simulink model "model_5LinkWalking"  (R2022b)
settings: Solver=ode45  StartTime=0.0  StopTime=Tf  FixedStep=1e-5  MaxStep=1e-3  RelTol=1e-12  AbsTol=1e-8
values from neighbouring files (symbols this model uses):
  des_traj_alpha = [ ... (first row only)    [main.m]
  f_dist = [0; -100; 0]    [main.m]
  gains = [ ... (first row only)    [main.m]
  gains_VSLIPSL = [gain_VSLIPSL.K_p; gain_VSLIPSL.K_d; gain_VSLIPSL.K_p_sw; gain_VSLIPSL.K_d_sw; gain_VSLIPSL.K_p_ds; gain_VSLIPSL.K_d_ds; gain_VSLIPSL.K_v_ds]    [main.m]
  init_flag = [1; 0; -dc.col_param.footPlus; -slipsl.time_ss(N); slipsl.x_ss(1); slipsl.y_ss(1); alpha_ss_ref(1)]    [main.m]
  Initial_state = [q0;dq0]    [main.m]
  param = [ ... (first row only)    [main.m]
  ref_star_ds = [ref_star.ds.x_CoM_star,      ref_star.ds.y_CoM_star, ref_star.ds.dx_CoM_star,      ref_star.ds.del_y_CoM_star, ref_star.ds.del_dx_CoM_star,      ref_star.ds.del2_y_CoM_star]    [main.m]
  ref_star_ss = [ref_star.ss.x_M_star,      ref_star.ss.y_M_star, ref_star.ss.x_swFoot_star, ref_star.ss.y_swFoot_star,      ref_star.ss.del_y_M_star, ref_star.ss.del_x_swFoot_star, ref_star.ss.del_y_swFoot_star,      ref_star.ss.del2_y_M_star, ref_star.ss.del2_x_swFoot_star, ref_star.ss.del2_y_swFoot_star,      ref_star.ss.x_CoM_star]    [main.m]
  sample_time = 0.001    [main.m]
  slipslParams = [ ... (first row only)    [main.m]
  slipslTraj_ds = [slipsl.time_ds, slipsl.x_ds, slipsl.y_ds, slipsl.dx_ds, slipsl.dy_ds, alpha_ds_ref_discrete]    [main.m]
  slipslTraj_ss = [slipsl.time_ss, slipsl.x_ss, slipsl.y_ss, slipsl.dx_ss, slipsl.dy_ss, alpha_ss_ref_discrete]    [main.m]
  swFootTraj = [swFootSLIPSL.x_CoM, swFootSLIPSL.x, swFootSLIPSL.z, swFootSLIPSL.dx, swFootSLIPSL.dz]    [main.m]
undefined symbols (not defined in the file or in its folder): sim_settings
libraries: simulink x1
(part 1 of 2)
settings Model: Creator=yamakita_lab  LastModifiedBy=mmpel
settings SolverCC: AutoScaleAbsTol=off  AlgebraicLoopSolver=TrustRegion
settings DataIOCC: ReturnWorkspaceOutputs=off
settings DebuggingCC: UnconnectedInputMsg=warning  UnconnectedOutputMsg=warning  UnconnectedLineMsg=warning  SFMachineParentedDataDiag=warning  ArithmeticOperatorsInVariantConditions=warning
settings ModelReferenceCC: EnableRefExpFcnMdlSchedulingChecks=on
settings SFSimCC: SimUseLocalCustomCode=off  CustomCodeUndefinedFunction=UseInterfaceOnly
settings RTWCC: RTWUseLocalCustomCode=off  DLArmComputeVersion=19.05

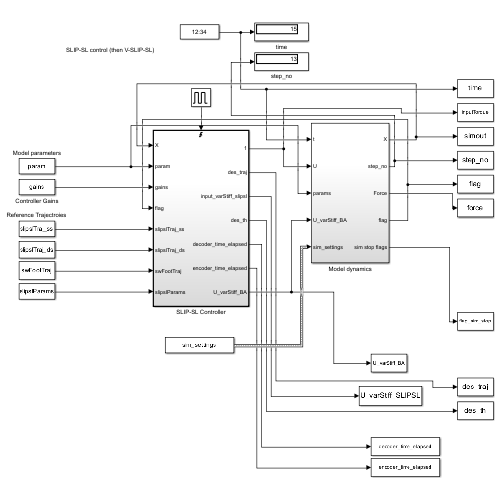
[thumbnail: Simulink's stored preview of the top-level diagram]
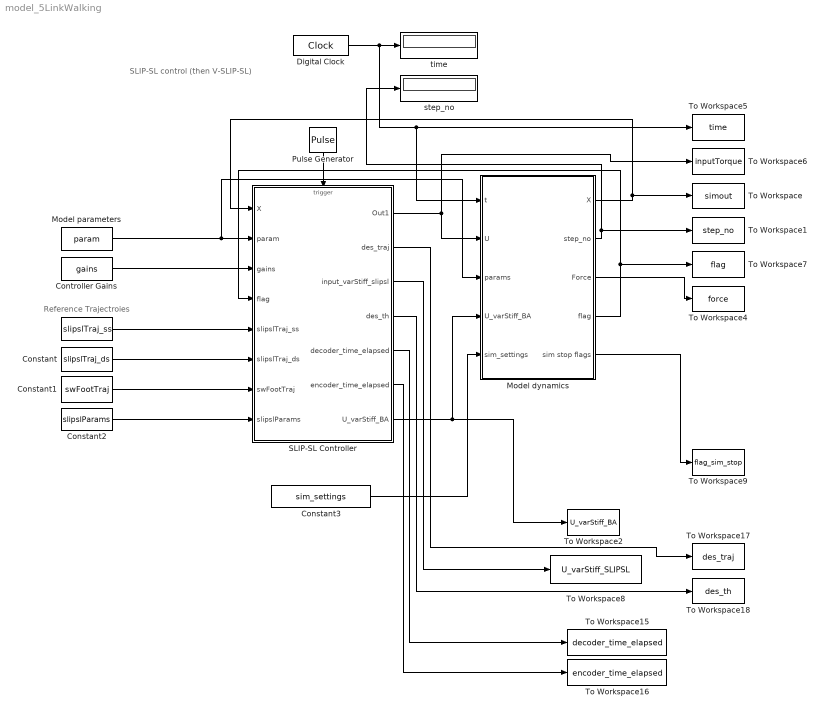
== system model_5LinkWalking ==
  note: Reference Trajectroies
  note: SLIP-SL control (then V-SLIP-SL)
  " " : Constant  Value=slipslTraj_ss
  Constant : Constant  Value=slipslTraj_ds
  Constant1 : Constant  Value=swFootTraj
  Constant2 : Constant  Value=slipslParams
  Constant3 : Constant  Value=sim_settings  VectorParams1D=off  OutDataTypeStr=Bus: sim_settings_bus
  Controller Gains : Constant  Value=gains
  Digital Clock : DigitalClock  SampleTime=1e-4
  Model dynamics : Subsystem
  Model parameters : Constant  Value=param  OutDataTypeStr=double
  Pulse Generator : DiscretePulseGenerator  PulseType=Time based  Period=5e-4  PulseWidth=5
  SLIP-SL Controller : Subsystem  TreatAsAtomicUnit=on
  To Workspace : ToWorkspace  VariableName=simout  SampleTime=sample_time
  To Workspace1 : ToWorkspace  VariableName=step_no  SampleTime=sample_time
  To Workspace15 : ToWorkspace  VariableName=decoder_time_elapsed  SampleTime=sample_time
  To Workspace16 : ToWorkspace  VariableName=encoder_time_elapsed  SampleTime=sample_time
  To Workspace17 : ToWorkspace  VariableName=des_traj  SampleTime=sample_time
  To Workspace18 : ToWorkspace  VariableName=des_th  SampleTime=sample_time
  To Workspace2 : ToWorkspace  VariableName=U_varStiff_BA  SampleTime=sample_time
  To Workspace4 : ToWorkspace  VariableName=force  SampleTime=sample_time
  To Workspace5 : ToWorkspace  VariableName=time  SampleTime=sample_time
  To Workspace6 : ToWorkspace  VariableName=inputTorque  SampleTime=sample_time
  To Workspace7 : ToWorkspace  VariableName=flag  SampleTime=sample_time
  To Workspace8 : ToWorkspace  VariableName=U_varStiff_SLIPSL  SampleTime=sample_time
  To Workspace9 : ToWorkspace  VariableName=flag_sim_stop  SampleTime=sample_time
  step_no : Display
  time : Display
  wires:
  SLIP-SL Controller/1(Out1) -> To Workspace6/1, Model dynamics/2(U)
  Model dynamics/1(X) -> SLIP-SL Controller/1(X), To Workspace/1
  Digital Clock/1 -> Model dynamics/1(t), To Workspace5/1, time/1
  Model dynamics/2(step_no) -> step_no/1, To Workspace1/1
  Model dynamics/3(Force) -> To Workspace4/1
  Model parameters/1 -> Model dynamics/3(params), SLIP-SL Controller/2(param)
  Controller Gains/1 -> SLIP-SL Controller/3(gains)
  Model dynamics/4(flag) -> To Workspace7/1, SLIP-SL Controller/4(flag)
  " "/1 -> SLIP-SL Controller/5(slipslTraj_ss)
  Constant1/1 -> SLIP-SL Controller/7(swFootTraj)
  Pulse Generator/1 -> SLIP-SL Controller/Trigger
  Model dynamics/5(sim stop flags) -> To Workspace9/1
  SLIP-SL Controller/3(input_varStiff_slipsl) -> To Workspace8/1
  SLIP-SL Controller/5(decoder_time_elapsed) -> To Workspace15/1
  SLIP-SL Controller/6(encoder_time_elapsed) -> To Workspace16/1
  SLIP-SL Controller/2(des_traj) -> To Workspace17/1
  SLIP-SL Controller/4(des_th) -> To Workspace18/1
  Constant/1 -> SLIP-SL Controller/6(slipslTraj_ds)
  Constant2/1 -> SLIP-SL Controller/8(slipslParams)
  SLIP-SL Controller/7(U_varStiff_BA) -> Model dynamics/4(U_varStiff_BA), To Workspace2/1
  Constant3/1 -> Model dynamics/5(sim_settings)

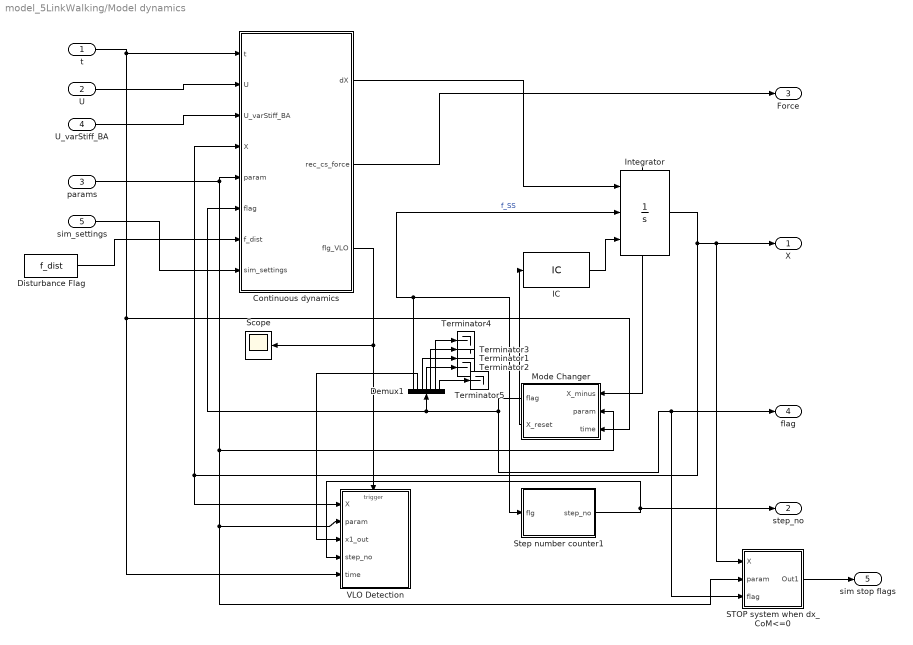
== system model_5LinkWalking/Model dynamics ==
  t : Inport
  U : Inport  Port=2
  params : Inport  Port=3
  U_varStiff_BA : Inport  Port=4
  sim_settings : Inport  Port=5
  Continuous dynamics : MATLAB Function  TreatAsAtomicUnit=on
  Demux1 : Demux  Outputs=7
  Disturbance Flag : Constant  Value=f_dist
  IC : InitialCondition  Value=Initial_state
  Integrator : Integrator  ExternalReset=falling  InitialConditionSource=external  ShowStatePort=on
  Mode Changer : Subsystem
  STOP system when dx_CoM<=0 : Subsystem
  Scope : Scope
  Step number counter1 : Subsystem
  Terminator{1..5} (5 alike) : Terminator
  VLO Detection : Subsystem  TreatAsAtomicUnit=on
  X : Outport  VectorParamsAs1DForOutWhenUnconnected=off
  step_no : Outport  Port=2  VectorParamsAs1DForOutWhenUnconnected=off
  Force : Outport  Port=3  VectorParamsAs1DForOutWhenUnconnected=off
  flag : Outport  Port=4
  sim stop flags : Outport  Port=5
  wires:
  IC/1 -> Integrator/3
  Integrator/State -> Mode Changer/1(X_minus)
  Continuous dynamics/1(dX) -> Integrator/1
  params/1 -> STOP system when dx_CoM<=0/2(param), VLO Detection/2(param), Mode Changer/2("param "), Continuous dynamics/5(param)
  U/1 -> Continuous dynamics/2(U)
  t/1 -> VLO Detection/5(time), Mode Changer/3(time), Continuous dynamics/1(t)
  Continuous dynamics/3(flg_VLO) -> Scope/1, VLO Detection/Trigger
  Integrator/1 -> STOP system when dx_CoM<=0/1(X), X/1, Continuous dynamics/4(X), VLO Detection/1(X)
  Mode Changer/2(X_reset) -> IC/1
  Mode Changer/1(flag) -> STOP system when dx_CoM<=0/3(flag), flag/1, Demux1/1, Continuous dynamics/6(flag)
  Demux1/2 -> VLO Detection/3(x1_out)
  Demux1/3 -> Terminator1/1
  Demux1/1 -> Step number counter1/1(flg), Integrator/2  "f_SS"
  Step number counter1/1(step_no) -> VLO Detection/4(step_no), step_no/1
  Continuous dynamics/2(rec_cs_force) -> Force/1
  Demux1/4 -> Terminator2/1
  Demux1/5 -> Terminator3/1
  Demux1/6 -> Terminator4/1
  STOP system when dx_CoM<=0/1(Out1) -> sim stop flags/1
  Disturbance Flag/1 -> Continuous dynamics/7(f_dist)
  Demux1/7 -> Terminator5/1
  U_varStiff_BA/1 -> Continuous dynamics/3(U_varStiff_BA)
  sim_settings/1 -> Continuous dynamics/8(sim_settings)

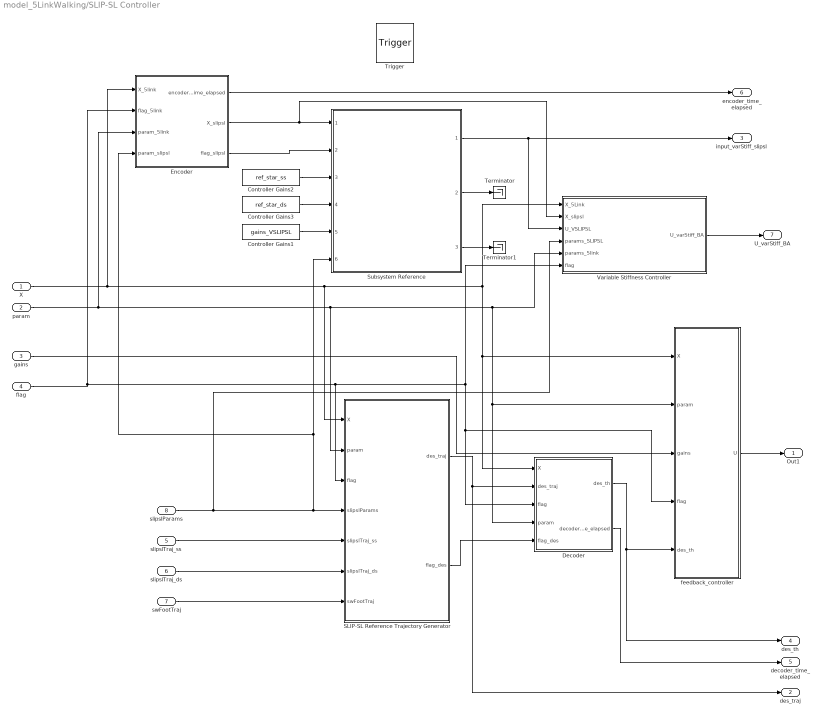
== system model_5LinkWalking/SLIP-SL Controller ==
  X : Inport
  param : Inport  Port=2
  gains : Inport  Port=3
  flag : Inport  Port=4
  slipslTraj_ss : Inport  Port=5
  slipslTraj_ds : Inport  Port=6
  swFootTraj : Inport  Port=7
  slipslParams : Inport  Port=8
  Trigger : TriggerPort  VariantControl=Variant  PortDimensions=1
  Controller Gains1 : Constant  Value=gains_VSLIPSL
  Controller Gains2 : Constant  Value=ref_star_ss
  Controller Gains3 : Constant  Value=ref_star_ds
  Decoder : MATLAB Function  TreatAsAtomicUnit=on
  Encoder : MATLAB Function  TreatAsAtomicUnit=on
  SLIP-SL Reference Trajectory Generator : MATLAB Function  TreatAsAtomicUnit=on
  Subsystem Reference : Subsystem  ReferencedSubsystem=VSLIPSL_controller_subsystem
  Terminator : Terminator
  Terminator1 : Terminator
  Variable Stiffness Controller : MATLAB Function  TreatAsAtomicUnit=on
  feedback_controller : MATLAB Function  TreatAsAtomicUnit=on
  Out1 : Outport  VectorParamsAs1DForOutWhenUnconnected=off
  des_traj : Outport  Port=2  InitialOutput=des_traj_alpha  VectorParamsAs1DForOutWhenUnconnected=off
  input_varStiff_slipsl : Outport  Port=3  VectorParamsAs1DForOutWhenUnconnected=off
  des_th : Outport  Port=4  PortDimensions=10  InitialOutput=Initial_state  VectorParamsAs1DForOutWhenUnconnected=off
  decoder_time_elapsed : Outport  Port=5  VectorParamsAs1DForOutWhenUnconnected=off
  encoder_time_elapsed : Outport  Port=6  VectorParamsAs1DForOutWhenUnconnected=off
  U_varStiff_BA : Outport  Port=7  VectorParamsAs1DForOutWhenUnconnected=off
  wires:
  feedback_controller/1(U) -> Out1/1
  X/1 -> SLIP-SL Reference Trajectory Generator/1(X), Variable Stiffness Controller/1(X_5Link), Decoder/1(X), feedback_controller/1(X), Encoder/1(X_5link)
  param/1 -> SLIP-SL Reference Trajectory Generator/2(param), Variable Stiffness Controller/5(params_5link), Decoder/4(param), feedback_controller/2(param), Encoder/3(param_5link)
  gains/1 -> feedback_controller/3(gains)
  flag/1 -> Encoder/2(flag_5link), Variable Stiffness Controller/6(flag), feedback_controller/4(flag), Decoder/3(flag), SLIP-SL Reference Trajectory Generator/3(flag)
  slipslTraj_ss/1 -> SLIP-SL Reference Trajectory Generator/5(slipslTraj_ss)
  swFootTraj/1 -> SLIP-SL Reference Trajectory Generator/7(swFootTraj)
  SLIP-SL Reference Trajectory Generator/1(des_traj) -> des_traj/1, Decoder/2(des_traj)
  slipslParams/1 -> Variable Stiffness Controller/4(params_SLIPSL), Encoder/4(param_slipsl), Subsystem Reference/6, SLIP-SL Reference Trajectory Generator/4(slipslParams)
  Controller Gains1/1 -> Subsystem Reference/5
  Controller Gains2/1 -> Subsystem Reference/3
  Controller Gains3/1 -> Subsystem Reference/4
  slipslTraj_ds/1 -> SLIP-SL Reference Trajectory Generator/6(slipslTraj_ds)
  Decoder/1(des_th) -> feedback_controller/5(des_th), des_th/1
  SLIP-SL Reference Trajectory Generator/2(flag_des) -> Decoder/5(flag_des)
  Decoder/2(decoder_time_elapsed) -> decoder_time_elapsed/1
  Encoder/2(X_slipsl) -> Variable Stiffness Controller/2(X_slipsl), Subsystem Reference/1
  Encoder/3(flag_slipsl) -> Subsystem Reference/2
  Subsystem Reference/2 -> Terminator/1
  Subsystem Reference/3 -> Terminator1/1
  Subsystem Reference/1 -> input_varStiff_slipsl/1, Variable Stiffness Controller/3(U_VSLIPSL)
  Encoder/1(encoder_time_elapsed) -> encoder_time_elapsed/1
  Variable Stiffness Controller/1(U_varStiff_BA) -> U_varStiff_BA/1

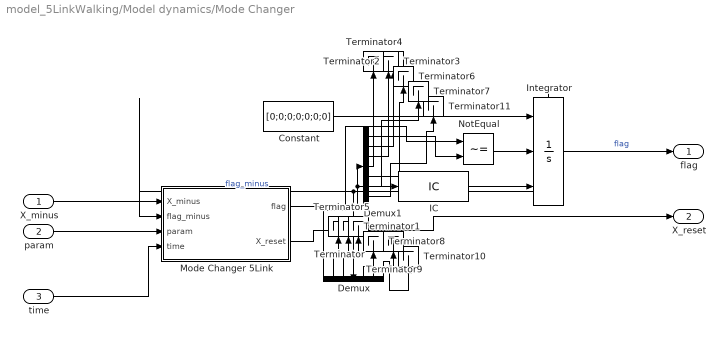
== system model_5LinkWalking/Model dynamics/Mode Changer ==
  X_minus : Inport
  "param " : Inport  Port=2
  time : Inport  Port=3
  Constant : Constant  Value=[0;0;0;0;0;0;0]
  Demux : Demux  Outputs=7
  Demux1 : Demux  Outputs=7
  IC : InitialCondition  Value=init_flag
  Integrator : Integrator  ExternalReset=rising  InitialConditionSource=external  ShowStatePort=on
  Mode Changer 5Link : MATLAB Function  TreatAsAtomicUnit=on
  NotEqual : RelationalOperator  Operator=~=  OutDataTypeStr=boolean  RndMeth=Simplest  InputSameDT=off
  Terminator{,1..11} (12 alike) : Terminator
  flag : Outport  VectorParamsAs1DForOutWhenUnconnected=off
  X_reset : Outport  Port=2  VectorParamsAs1DForOutWhenUnconnected=off
  wires:
  X_minus/1 -> Mode Changer 5Link/1(X_minus)
  IC/1 -> Integrator/3
  Integrator/State -> Mode Changer 5Link/2(flag_minus), Demux/1  "flag_minus"
  "param "/1 -> Mode Changer 5Link/3(param)
  Mode Changer 5Link/1(flag) -> Demux1/1, IC/1
  Constant/1 -> Integrator/1
  NotEqual/1 -> Integrator/2
  Integrator/1 -> flag/1  "flag"
  Mode Changer 5Link/2(X_reset) -> X_reset/1
  Demux/1 -> NotEqual/1
  Demux/3 -> Terminator1/1
  Demux/2 -> Terminator/1
  Demux1/1 -> NotEqual/2
  Demux1/2 -> Terminator2/1
  Demux1/3 -> Terminator3/1
  time/1 -> Mode Changer 5Link/4(time)
  Demux1/4 -> Terminator4/1
  Demux/4 -> Terminator5/1
  Demux/5 -> Terminator8/1
  Demux/6 -> Terminator9/1
  Demux1/5 -> Terminator6/1
  Demux1/6 -> Terminator7/1
  Demux/7 -> Terminator10/1
  Demux1/7 -> Terminator11/1

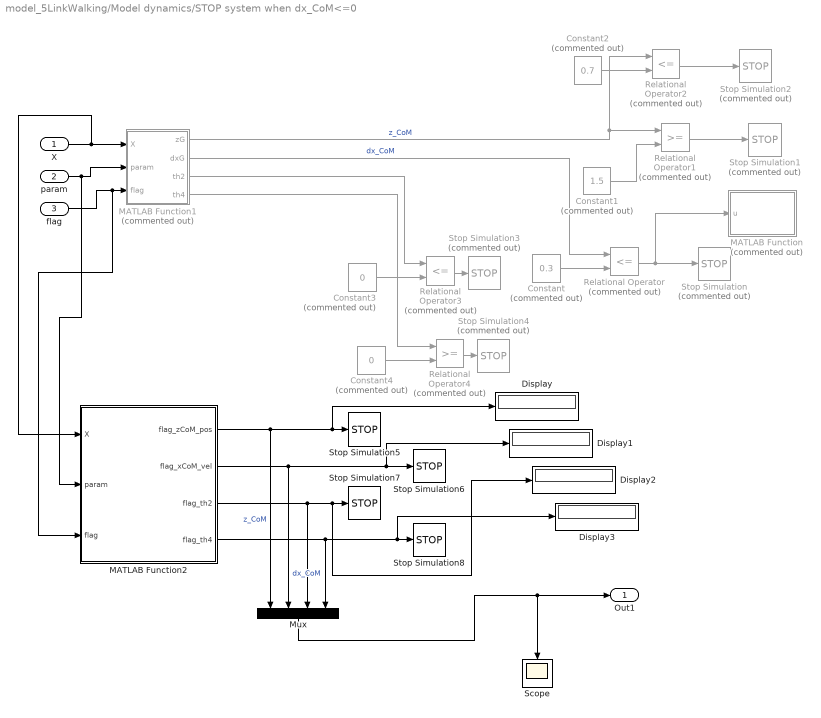
== system model_5LinkWalking/Model dynamics/STOP system when dx_CoM<=0 ==
  X : Inport
  param : Inport  Port=2
  flag : Inport  Port=3
  Constant : Constant  Commented=on  Value=0.3
  Constant1 : Constant  Commented=on  Value=1.5
  Constant2 : Constant  Commented=on  Value=0.7
  Constant3 : Constant  Commented=on  Value=0
  Constant4 : Constant  Commented=on  Value=0
  Display{,1..3} (4 alike) : Display
  MATLAB Function : MATLAB Function  Commented=on  TreatAsAtomicUnit=on
  MATLAB Function1 : MATLAB Function  Commented=on  TreatAsAtomicUnit=on
  MATLAB Function2 : MATLAB Function  TreatAsAtomicUnit=on
  Mux : Mux
  Relational Operator : RelationalOperator  Commented=on  Operator=<=  OutDataTypeStr=boolean  RndMeth=Simplest  InputSameDT=off
  Relational Operator1 : RelationalOperator  Commented=on  OutDataTypeStr=boolean  RndMeth=Simplest  InputSameDT=off
  Relational Operator2 : RelationalOperator  Commented=on  Operator=<=  OutDataTypeStr=boolean  RndMeth=Simplest  InputSameDT=off
  Relational Operator3 : RelationalOperator  Commented=on  Operator=<=  OutDataTypeStr=boolean  RndMeth=Simplest  InputSameDT=off
  Relational Operator4 : RelationalOperator  Commented=on  OutDataTypeStr=boolean  RndMeth=Simplest  InputSameDT=off
  Scope : Scope
  Stop Simulation{,1..4} (5 alike) : Stop  Commented=on
  Stop Simulation{5..8} (4 alike) : Stop
  Out1 : Outport
  wires:
  Constant/1 -> Relational Operator/2
  Relational Operator/1 -> Stop Simulation/1, MATLAB Function/1(u)
  MATLAB Function1/2(dxG) -> Relational Operator/1  "dx_CoM"
  MATLAB Function1/1(zG) -> Relational Operator2/1, Relational Operator1/1  "z_CoM"
  Relational Operator1/1 -> Stop Simulation1/1
  Constant1/1 -> Relational Operator1/2
  Relational Operator2/1 -> Stop Simulation2/1
  Constant2/1 -> Relational Operator2/2
  X/1 -> MATLAB Function2/1(X), MATLAB Function1/1(X)
  param/1 -> MATLAB Function2/2(param), MATLAB Function1/2(param)
  flag/1 -> MATLAB Function2/3(flag), MATLAB Function1/3(flag)
  MATLAB Function1/3(th2) -> Relational Operator3/1
  Constant3/1 -> Relational Operator3/2
  MATLAB Function1/4(th4) -> Relational Operator4/1
  Constant4/1 -> Relational Operator4/2
  Relational Operator3/1 -> Stop Simulation3/1
  Relational Operator4/1 -> Stop Simulation4/1
  MATLAB Function2/1(flag_zCoM_pos) -> Mux/1, Display/1, Stop Simulation5/1  "z_CoM"
  MATLAB Function2/2(flag_xCoM_vel) -> Mux/2, Display1/1, Stop Simulation6/1  "dx_CoM"
  MATLAB Function2/3(flag_th2) -> Display2/1, Stop Simulation7/1, Mux/3
  MATLAB Function2/4(flag_th4) -> Mux/4, Display3/1, Stop Simulation8/1
  Mux/1 -> Scope/1, Out1/1

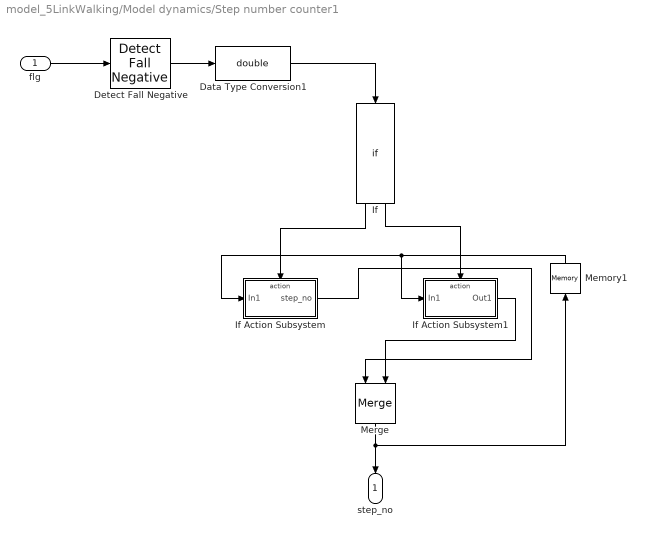
== system model_5LinkWalking/Model dynamics/Step number counter1 ==
  flg : Inport  SampleTime=sample_time
  Data Type Conversion1 : DataTypeConversion  OutDataTypeStr=double  SaturateOnIntegerOverflow=off  RndMeth=Floor
  Detect Fall Negative : simulink/Logic and Bit Operations/Detect Fall Negative  vinit=0  OutDataTypeStr=boolean
  If : If
  If Action Subsystem : Subsystem  TreatAsAtomicUnit=on
  If Action Subsystem1 : Subsystem  TreatAsAtomicUnit=on
  Memory1 : Memory
  Merge : Merge  InitialOutput=0
  step_no : Outport  VectorParamsAs1DForOutWhenUnconnected=off
  wires:
  flg/1 -> Detect Fall Negative/1
  If/1 -> If Action Subsystem/Action
  If Action Subsystem/1(step_no) -> Merge/1
  If Action Subsystem1/1(Out1) -> Merge/2
  If/2 -> If Action Subsystem1/Action
  Memory1/1 -> If Action Subsystem/1(In1), If Action Subsystem1/1(In1)
  Data Type Conversion1/1 -> If/1
  Detect Fall Negative/1 -> Data Type Conversion1/1
  Merge/1 -> Memory1/1, step_no/1

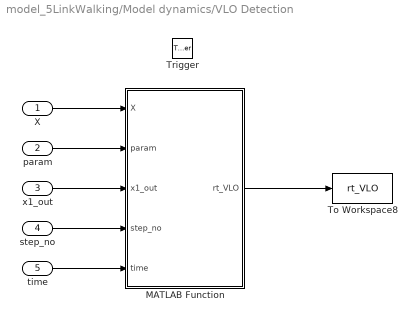
== system model_5LinkWalking/Model dynamics/VLO Detection ==
  X : Inport
  param : Inport  Port=2
  x1_out : Inport  Port=3
  step_no : Inport  Port=4
  time : Inport  Port=5
  Trigger : TriggerPort  VariantControl=Variant
  MATLAB Function : MATLAB Function  TreatAsAtomicUnit=on
  To Workspace8 : ToWorkspace  VariableName=rt_VLO  SampleTime=-1
  wires:
  X/1 -> MATLAB Function/1(X)
  MATLAB Function/1(rt_VLO) -> To Workspace8/1
  param/1 -> MATLAB Function/2(param)
  x1_out/1 -> MATLAB Function/3(x1_out)
  step_no/1 -> MATLAB Function/4(step_no)
  time/1 -> MATLAB Function/5(time)

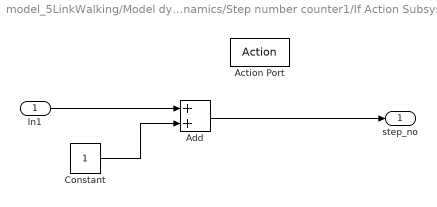
== system model_5LinkWalking/Model dynamics/Step number counter1/If Action Subsystem ==
  In1 : Inport
  Action Port : ActionPort  ActionPortLabel=if(u1 > 0)
  Add : Sum
  Constant : Constant
  step_no : Outport
  wires:
  In1/1 -> Add/1
  Constant/1 -> Add/2
  Add/1 -> step_no/1

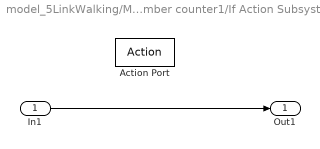
== system model_5LinkWalking/Model dynamics/Step number counter1/If Action Subsystem1 ==
  In1 : Inport
  Action Port : ActionPort  ActionPortLabel=else
  Out1 : Outport
  wires:
  In1/1 -> Out1/1

== matlab function model_5LinkWalking/Model dynamics/Mode Changer/Mode Changer 5Link ==
  data: X_minus input; flag output; flag_minus input; param input; X_reset output; time input
function [flag, X_reset]  = fcn(X_minus, flag_minus, param, time)

%% variables

th1 = X_minus(1);
th2 = X_minus(2);
th3 = X_minus(3);
th4 = X_minus(4);
th5 = X_minus(5);

dth1 = X_minus(6);
dth2 = X_minus(7);
dth3 = X_minus(8);
dth4 = X_minus(9);
dth5 = X_minus(10);

q = [th1;th2;th3;th4;th5];
dq = [dth1;dth2;dth3;dth4;dth5];

%% parameters

m1 = param(1);
m2 = param(2);
m3 = m2;
m4 = m1;
m5 = param(3);

l1 = param(4);
l2 = param(5);
l5 = param(6);
l3 = l2;
l4 = l1;

gravi = param(7);
I1 = param(8);
I2 = param(9);
I5 = param(10);
I3 = I1;
I4 = I2;

q_minus = [th1;th2;th3;th4;th5];
dq_minus = [dth1;dth2;dth3;dth4;dth5];

%% flags
f_SS = flag_minus(1); % indicates which stance phase it is
foot = flag_minus(2); % location of the stance foot
foot_prev = flag_minus(3); % previous location of the stance foot
% time = flag_minus(4); % previous location of the stance foot
x_LO = flag_minus(5); % x_CoM location when liftOff happens
z_LO = flag_minus(6); % z_CoM location when liftOff happens

%%
X_reset = [q_minus; dq_minus]; % dummy X_reset so that simulink doesn't give error

%% calculating the Swing foot position and velocity
Psw_tip_minus = [l1*cos(th1) + l2*cos(th1 + th2) + l3*cos(th1 + th2 + th3) + l4*cos(th1 + th2 + th3 + th4);
                 l1*sin(th1) + l2*sin(th1 + th2) + l3*sin(th1 + th2 + th3) + l4*sin(th1 + th2 + th3 + th4)];
 
J_Psw_tip_minus = [- l4*sin(th1 + th2 + th3 + th4) - l2*sin(th1 + th2) - l1*sin(th1) - l3*sin(th1 + th2 + th3), - l4*sin(th1 + th2 + th3 + th4) - l2*sin(th1 + th2) - l3*sin(th1 + th2 + th3), - l4*sin(th1 + th2 + th3 + th4) - l3*sin(th1 + th2 + th3), -l4*sin(th1 + th2 + th3 + th4), 0;
                   l4*cos(th1 + th2 + th3 + th4) + l2*cos(th1 + th2) + l1*cos(th1) + l3*cos(th1 + th2 + th3),   l4*cos(th1 + th2 + th3 + th4) + l2*cos(th1 + th2) + l3*cos(th1 + th2 + th3),   l4*cos(th1 + th2 + th3 + th4) + l3*cos(th1 + th2 + th3),  l4*cos(th1 + th2 + th3 + th4), 0];

dPsw_tip_minus = J_Psw_tip_minus*dq_minus;

%%
if f_SS == 1 && Psw_tip_minus(2,1) <= 0 && ( ( Psw_tip_minus(1,1) > 0 && dPsw_tip_minus(2,1) <= 0) || ( Psw_tip_minus(1,1) <= 0 && dPsw_tip_minus(2,1) <= -0.5) )
    % change from single stance phase to double stance phase
    f_SS = -1;
    foot_prev = foot; % saving the old foot location
    foot = foot_prev + Psw_tip_minus(1,1); % calculating the new foots location
           
    % Impact mapによる衝突後の状態の計算
    MM_minus = MM_matrix(X_minus,param);
    dq_after = (eye(5)-inv(MM_minus)*J_Psw_tip_minus'*inv(J_Psw_tip_minus*inv(MM_minus)*J_Psw_tip_minus')*J_Psw_tip_minus)*dq_minus;

    th1_after = q_minus(4,1) + q_minus(3,1) + q_minus(2,1) + q_minus(1,1) - pi; % th1 becomes th4
    th2_after = - q_minus(4,1); % th2 becomes th3
    th3_after = - q_minus(3,1); % th3 becomes th2
    th4_after = - q_minus(2,1); % th4 becomes th1
    th5_after = q_minus(5,1) - q_minus(3,1) + pi;
    
    q_after = [th1_after; th2_after; th3_after; th4_after; th5_after]; % this is where the switching happens
    
    dth1_after = dq_after(4,1) + dq_after(3,1) + dq_after(2,1) + dq_after(1,1); % th1 becomes th4
    dth2_after = - dq_after(4,1); % th2 becomes th3
    dth3_after = - dq_after(3,1); % th3 becomes th2
    dth4_after = - dq_after(2,1); % th4 becomes th1
    dth5_after = dq_after(5,1) - dq_after(3,1) ;
    
    % Reset state if the f_ss change from 1 to 0 (from single stance to
    % double stance)
    X_reset = [q_after; dth1_after; dth2_after; dth3_after; dth4_after; dth5_after];

elseif f_SS == -1 && dPsw_tip_minus(2,1) > 0.005
    % change from double stance phase to single stance phase if the y
    % component of the contraint force becomes negative
    f_SS = 1;
    % reset X to restart swing leg with zero initial velocity from the
    % position that swing leg last was
    X_reset = X_minus;
    
    % calculating CoM pos
    CoM = calculate_com(X_minus, param, foot, [0;0;0;0;0]);
    x_LO = CoM(1);
    z_LO = CoM(2);        
end
alpha_LO = pi - (2*th1 + th2)/2;
flag = [f_SS; foot; foot_prev; time; x_LO; z_LO; alpha_LO];

== matlab function model_5LinkWalking/Model dynamics/STOP system when dx_CoM<=0/MATLAB Function2 ==
  data: X input; param input; flag input; flag_zCoM_pos output; flag_xCoM_vel output; flag_th2 output; flag_th4 output
function [flag_zCoM_pos, flag_xCoM_vel, flag_th2, flag_th4] = fcn(X,param, flag)

%% variables
th1 = X(1);
th2 = X(2);
th3 = X(3);
th4 = X(4);
th5 = X(5);

dth1 = X(6);
dth2 = X(7);
dth3 = X(8);
dth4 = X(9);
dth5 = X(10);

q = [th1;th2;th3;th4;th5];
dq = [dth1;dth2;dth3;dth4;dth5];

%% parameters

m1 = param(1);
m2 = param(2);
m3 = m2;
m4 = m1;
m5 = param(3);

l1 = param(4);
l2 = param(5);
l5 = param(6);
l3 = l2;
l4 = l1;

gravi = param(7);
I1 = param(8);
I2 = param(9);
I5 = param(10);
I3 = I1;
I4 = I2;

%% flags
f_SS = flag(1); % indicates which stance phase it is
foot = flag(2); % location of the stance foot
foot_prev = flag(3); % previous location of the stance foot

%% CoM calculation
% CoM = [xG, zG, dxG, dzG, ddxG, ddzG];
CoM = calculate_com(X, param, 0, [0;0;0;0;0]); % calculation the CoM location

xG = CoM(1);
zG = CoM(2);
dxG = CoM(3);
dzG = CoM(4);

%%

% flag_zCoM_pos: if z_CoM drops or rises above certain value
flag_zCoM_pos = 0;
if zG >= 1.5
    flag_zCoM_pos = 1;
elseif zG <= 0.7
    flag_zCoM_pos = 1;
end

% flag_xCoM_vel
flag_xCoM_vel = 0;
% if dxG <= 0
%     flag_xCoM_vel = 1;
% end

% flag_th2
flag_th2 = 0;
if mod(th2, 2*pi) <= 0
    flag_th2 = 1;
end

% flag_th4
flag_th4 = 0;
if th4 >= 0
%     flag_th4 = 1;
end

== matlab function model_5LinkWalking/SLIP-SL Controller/SLIP-SL Reference Trajectory Generator ==
  data: des_traj output; X input; param input; flag input; slipslParams input; slipslTraj_ss input; slipslTraj_ds input; swFootTraj input; flag_des output
function [des_traj, flag_des] = fcn( ...
    X, param, flag, slipslParams, slipslTraj_ss, slipslTraj_ds, swFootTraj)

%% variables
th1 = X(1);
th2 = X(2);
th3 = X(3);
th4 = X(4);
th5 = X(5);

dth1 = X(6);
dth2 = X(7);
dth3 = X(8);
dth4 = X(9);
dth5 = X(10);

q = [th1;th2;th3;th4;th5];
dq = [dth1;dth2;dth3;dth4;dth5];

%% flags
f_SS = flag(1); % indicates which stance phase it is
foot = flag(2); % location of the stance foot
foot_prev = flag(3); % previous location of the stance foot

t_mode_change = flag(4); % time stamp when the mode change happens (TD or LO)

x_LO = flag(5); % lift off location of CoM when it happened
alpha_mode_change = flag(7); % lift off location of CoM when it happened

%% CoM desired position and velocity calculation

time_ss = slipslTraj_ss(:,1);
x_slip_ss = slipslTraj_ss(:,2);
y_slip_ss = slipslTraj_ss(:,3);
dx_slip_ss = slipslTraj_ss(:,4);
dy_slip_ss = slipslTraj_ss(:,5);
alpha_ss = slipslTraj_ss(:,6);

time_ds = slipslTraj_ds(:,1);
x_slip_ds = slipslTraj_ds(:,2);
y_slip_ds = slipslTraj_ds(:,3);
dx_slip_ds = slipslTraj_ds(:,4);
dy_slip_ds = slipslTraj_ds(:,5);
alpha_ds = slipslTraj_ds(:,6);

CoM = calculate_com(X, param, foot, [0;0;0;0;0]); % calculating the location of CoM

x_CoM = CoM(1) - flag(2);

%% alpha based ref. traj. generation
alpha = wrapTo2Pi(pi - (2*X(1) + X(2))/2);
alpha_curr_step = alpha;
% alpha_curr_step = alpha - alpha_mode_change; % relative alpha TODO: 
% get rid off this and do the alpha merge thing I did in AIM2022 paper.

if f_SS == 1
    % if we are in the SS phase
    
    % CoM Trajectory
    if alpha_curr_step <= alpha_ss(end)
        % if the current time is within the SLIP-SL SS time
        
        x_CoM_alpha_des = interp1(alpha_ss, x_slip_ss, alpha_curr_step);
        y_CoM_alpha_des = interp1(alpha_ss, y_slip_ss, alpha_curr_step);
        dx_CoM_alpha_des = interp1(alpha_ss, dx_slip_ss, alpha_curr_step);
        dy_CoM_alpha_des = interp1(alpha_ss, dy_slip_ss, alpha_curr_step);

        x_sw_alpha_des = interp1(alpha_ss, swFootTraj(:,2), alpha_curr_step);
        y_sw_alpha_des = interp1(alpha_ss, swFootTraj(:,3), alpha_curr_step);
        dx_sw_alpha_des = interp1(alpha_ss, swFootTraj(:,4), alpha_curr_step);
        dy_sw_alpha_des = interp1(alpha_ss, swFootTraj(:,5), alpha_curr_step);
        
        flag_des = 1; % desired stance of the robot according to the slip traj
    else
        % if the current time has passed the time defined in SLIP-SL traj
        % (i.e. transition to DS is late)
        
        x_CoM_alpha_des = x_CoM; % current position of the x_CoM
        y_CoM_alpha_des = y_slip_ss(end);
        dx_CoM_alpha_des = dx_slip_ss(end);
        dy_CoM_alpha_des = dy_slip_ss(end);

        x_sw_alpha_des = swFootTraj(end,2);
        y_sw_alpha_des = swFootTraj(end,3);
        dx_sw_alpha_des = swFootTraj(end,4);
        dy_sw_alpha_des = swFootTraj(end,5) - 0.5*(alpha_curr_step - alpha_ss(end));
        
        flag_des = 2; % desired stance of the robot according to the slip traj
    end
    
else
    % if we are in the DS phase

    % CoM Trajectory    
    footPlus = slipslParams(18); % position of footPlus for reference traj
    
    if alpha_curr_step <= alpha_ds(1)
        % TODO: write definition
        
        x_CoM_alpha_des = x_slip_ds(1) - footPlus;
        y_CoM_alpha_des = y_slip_ds(1);
        dx_CoM_alpha_des = dx_slip_ds(1);
        dy_CoM_alpha_des = dy_slip_ds(1);
        
        flag_des = 2; % desired stance of the robot according to the slip traj

    elseif alpha_curr_step <= alpha_ds(end)
        % if the current time is within the SLIP-SL DS time
        
        x_CoM_alpha_des = interp1(alpha_ds, x_slip_ds, alpha_curr_step) - footPlus;
        y_CoM_alpha_des = interp1(alpha_ds, y_slip_ds, alpha_curr_step);
        dx_CoM_alpha_des = interp1(alpha_ds, dx_slip_ds, alpha_curr_step);
        dy_CoM_alpha_des = interp1(alpha_ds, dy_slip_ds, alpha_curr_step);
        
        flag_des = 2; % desired stance of the robot according to the slip traj
    else
        % if the current time has passed the time defined in SLIP-SL traj
        % (i.e. transition to SS is late)

        x_CoM_alpha_des = x_slip_ds(end) - footPlus;
        y_CoM_alpha_des = y_slip_ds(end);
        dx_CoM_alpha_des = dx_slip_ds(end);
        dy_CoM_alpha_des = dy_slip_ds(end);
        
        flag_des = 1; % desired stance of the robot according to the slip traj
    end
    
    % Swing Foot Trajectory
    x_sw_alpha_des = foot_prev;
    y_sw_alpha_des = 0;
    dx_sw_alpha_des = 0;
    dy_sw_alpha_des = 0;
end

%% outputs
flag_des = flag_des;

%% finding the desired joint angles

des_traj = [
    x_CoM_alpha_des; y_CoM_alpha_des; x_sw_alpha_des; y_sw_alpha_des;
    dx_CoM_alpha_des; dy_CoM_alpha_des; dx_sw_alpha_des; dy_sw_alpha_des];

== matlab function model_5LinkWalking/SLIP-SL Controller/Decoder ==
  data: X input; des_th output; des_traj input; flag input; param input; flag_des input; decoder_time_elapsed output
function [des_th, decoder_time_elapsed] = fcn(X, des_traj, flag, param, flag_des)

% debug
if flag(1) == 1
    xd = 0;
else
    xd = 0;
end

 % assume stance foot is at x = 0
flag(3) = flag(3) - flag(2);
flag(2) = 0;

[des_th, decoder_time_elapsed] = calc_desJointAngles(X, des_traj, flag, param, flag_des);

== matlab function model_5LinkWalking/SLIP-SL Controller/Encoder ==
  data: encoder_time_elapsed output; X_5link input; X_slipsl output; flag_slipsl output; flag_5link input; param_5link input; param_slipsl input
function [encoder_time_elapsed, X_slipsl, flag_slipsl] = fcn(X_5link, flag_5link, param_5link, param_slipsl)

%% variables
th1 = X_5link(1);
th2 = X_5link(2);
th3 = X_5link(3);
th4 = X_5link(4);
th5 = X_5link(5);

dth1 = X_5link(6);
dth2 = X_5link(7);
dth3 = X_5link(8);
dth4 = X_5link(9);
dth5 = X_5link(10);

q = [th1;th2;th3;th4;th5];
dq = [dth1;dth2;dth3;dth4;dth5];

%% flags
f_SS = flag_5link(1); % indicates which stance phase it is
foot = flag_5link(2); % location of the stance foot
foot_prev = flag_5link(3); % previous location of the stance foot

t_mode_change = flag_5link(4); % time stamp when the mode change happens (TD or LO)

x_LO = flag(5); % lift off location of CoM when it happened
alpha_mode_change = flag_5link(7); % lift off location of CoM when it happened

X_slipsl_ss = NaN(8,1);

encoder_time_elapsed = NaN;

%%
foot_relative = 0;
CoM = calculate_com(X_5link, param_5link, foot_relative, [0;0;0;0;0]); % calculating the location of CoM
x_CoM = CoM(1);
y_CoM = CoM(2);

dx_CoM = CoM(3);
dy_CoM = CoM(4);

if f_SS == 1
    [X_slipsl_ss, encoder_time_elapsed] = calc_5linkTOslipsl(X_5link, flag_5link, param_5link, param_slipsl);
end

X_slipsl = [
    X_slipsl_ss(1:4); x_CoM; y_CoM;
    X_slipsl_ss(5:8); dx_CoM; dy_CoM;
    ];

flag_slipsl = [f_SS; 0; foot_prev - foot];

end

== matlab function model_5LinkWalking/SLIP-SL Controller/Variable Stiffness Controller ==
  data: X_5Link input; X_slipsl input; U_VSLIPSL input; U_varStiff_BA output; params_SLIPSL input; params_5link input; flag input
function U_varStiff_BA  = fcn(X_5Link, X_slipsl, U_VSLIPSL, params_SLIPSL,  params_5link, flag)

%% SLIP-SL constant params

L0_ss = params_SLIPSL(1); % [m]
k0_ss = params_SLIPSL(2); % nominal leg stiffness [N/m]
m_M = params_SLIPSL(3); % hip mass [kg]
m_swLeg = params_SLIPSL(4); % [kg]
m_swFoot = params_SLIPSL(5); % [kg]
I_swLeg = params_SLIPSL(6); %
I_swFoot = params_SLIPSL(7); %
L_thigh = params_SLIPSL(8); % [m]
k_swFoot = params_SLIPSL(9); %
k_swLeg = params_SLIPSL(10); %
theta0 = params_SLIPSL(11); %[rad]
r0 = params_SLIPSL(12); % [m]
gravi = params_SLIPSL(13); % gravitational acc

L0_ds = params_SLIPSL(14); % [m] free length of the springs in the DS
k0_ds = params_SLIPSL(15); % [N/m] stiffness of the springs in the DS

bound_cst = params_SLIPSL(16); % clipped = max(min(x, upper), lower);

%% 5-link model parameters

m1 = params_5link(1);
m2 = params_5link(2);
m3 = m2;
m4 = m1;
m5 = params_5link(3);

l1 = params_5link(4);
l2 = params_5link(5);
l5 = params_5link(6);
l3 = l2;
l4 = l1;

gravi = params_5link(7);
I1 = params_5link(8);
I2 = params_5link(9);
I5 = params_5link(10);
I3 = I1;
I4 = I2;

r_k = params_5link(11);
r_h = params_5link(12);
k_ba = params_5link(13);
phi_h0 = params_5link(14);
phi_k0 = params_5link(15);

varStiff_control_reduction_ratio = params_5link(16);

%% flag

f_SS = flag(1); % indicates which stance phase it is
foot = flag(2); % location of the stance foot
foot_prev = flag(3); % previous location of the stance foot

t_mode_change = flag(4); % time stamp when the mode change happens (TD or LO)

x_LO = flag(5); % lift off location of CoM when it happened
alpha_mode_change = flag(7); % lift off location of CoM when it happened

%% SLIPSL State - Already normalized wrt. stance foot location

x_M = X_slipsl(1); % x position of main mass in SS
y_M = X_slipsl(2); % z position of main mass in SS
theta = X_slipsl(3); % angle of the swing leg when in SS
r = X_slipsl(4); % distance of the foot from the knee on SS
x_CoM = X_slipsl(5);% x position of the CoM
y_CoM = X_slipsl(6);

dx_M = X_slipsl(7); % x velocity of main mass in SS
dy_M = X_slipsl(8); % z velocity of main mass in SS
dtheta = X_slipsl(9);
dr = X_slipsl(10);
dx_CoM = X_slipsl(11);
dy_CoM = X_slipsl(12);

%% Variable stiffness controller
% Derivation: OneNote/Research Diary (Doctor)/Variable BA stiffness

if f_SS == 1
    % Single stance phase
    
    ratio_var_stiff = (k0_ss + U_VSLIPSL(1))/k0_ss;
    u_st = varStiff_control_reduction_ratio*(ratio_var_stiff - 1)*k_ba;
    
    PE_nominal_SLIPSL_sw = 0.5*k_swLeg*(theta0 - theta)^2 ...
        + 0.5*k_swFoot*(r0 - r)^2;
    PE_varStiff_SLIPSL_sw = 0.5*(k_swLeg + U_VSLIPSL(2))*(theta0 - theta)^2 ...
        + 0.5*(k_swFoot + U_VSLIPSL(3))*(r0 - r)^2;
    ratio_var_stiff_sw = PE_varStiff_SLIPSL_sw/PE_nominal_SLIPSL_sw;
    u_sw = varStiff_control_reduction_ratio*(ratio_var_stiff_sw - 1)*k_ba;
else
    % Double stance phase
    
    ratio_var_stiff_st = (k0_ds + U_VSLIPSL(4))/k0_ds;
    ratio_var_stiff_sw = (k0_ds + U_VSLIPSL(5))/k0_ds;

    u_st = varStiff_control_reduction_ratio*(ratio_var_stiff_st - 1)*k_ba;
    u_sw = varStiff_control_reduction_ratio*(ratio_var_stiff_sw - 1)*k_ba;
end


U_varStiff_BA = [u_st; u_sw];

== matlab function model_5LinkWalking/Model dynamics/STOP system when dx_CoM<=0/MATLAB Function ==
  data: u input
function fcn(u)
if u ~= 0
    disp('dx < 0')
end

== matlab function model_5LinkWalking/Model dynamics/Continuous dynamics ==
  data: t input; U input; U_varStiff_BA input; dX output; rec_cs_force output; X input; param input; flg_VLO output; flag input; f_dist input; sim_settings input Bus: sim_settings_bus
function [dX, rec_cs_force, flg_VLO] = fcn(t, U, U_varStiff_BA, X, param, flag, f_dist, sim_settings)

%% variables
th1 = X(1);
th2 = X(2);
th3 = X(3);
th4 = X(4);
th5 = X(5);

dth1 = X(6);
dth2 = X(7);
dth3 = X(8);
dth4 = X(9);
dth5 = X(10);

q = [th1;th2;th3;th4;th5];
dq = [dth1;dth2;dth3;dth4;dth5];

%% parameters

m1 = param(1);
m2 = param(2);
m3 = m2;
m4 = m1;
m5 = param(3);

l1 = param(4);
l2 = param(5);
l5 = param(6);
l3 = l2;
l4 = l1;

gravi = param(7);
I1 = param(8);
I2 = param(9);
I5 = param(10);
I3 = I1;
I4 = I2;

r_k = param(11);
r_h = param(12);
k_ba = param(13);
phi_h0 = param(14);
phi_k0 = param(15);

%% flags
f_SS = flag(1); % indicates which stance phase it is
foot = flag(2); % location of the stance foot
foot_prev = flag(3); % previous location of the stance foot

%% Inertia Matrix
MM = MM_matrix(X,param);

%% Centrifugal force · Coriolis force Vector
CC = zeros(5,1);

CC(1, 1) = - (dth2^2*l1*l3*m3*sin(th2 + th3))/2 - dth2^2*l1*l3*m4*sin(th2 + th3) - (dth3^2*l1*l3*m3*sin(th2 + th3))/2 - dth3^2*l1*l3*m4*sin(th2 + th3) - (dth2^2*l1*l5*m5*sin(th2 + th5))/2 - (dth3^2*l2*l4*m4*sin(th3 + th4))/2 - (dth4^2*l2*l4*m4*sin(th3 + th4))/2 - (dth5^2*l1*l5*m5*sin(th2 + th5))/2 - (dth2^2*l1*l2*m2*sin(th2))/2 - dth2^2*l1*l2*m3*sin(th2) - dth2^2*l1*l2*m4*sin(th2) - dth2^2*l1*l2*m5*sin(th2) - (dth3^2*l2*l3*m3*sin(th3))/2 - dth3^2*l2*l3*m4*sin(th3) - (dth4^2*l3*l4*m4*sin(th4))/2 - (dth5^2*l2*l5*m5*sin(th5))/2 - (dth2^2*l1*l4*m4*sin(th2 + th3 + th4))/2 - (dth3^2*l1*l4*m4*sin(th2 + th3 + th4))/2 - (dth4^2*l1*l4*m4*sin(th2 + th3 + th4))/2 - dth1*dth2*l1*l3*m3*sin(th2 + th3) - 2*dth1*dth2*l1*l3*m4*sin(th2 + th3) - dth1*dth3*l1*l3*m3*sin(th2 + th3) - 2*dth1*dth3*l1*l3*m4*sin(th2 + th3) - dth2*dth3*l1*l3*m3*sin(th2 + th3) - 2*dth2*dth3*l1*l3*m4*sin(th2 + th3) - dth1*dth2*l1*l5*m5*sin(th2 + th5) - dth1*dth3*l2*l4*m4*sin(th3 + th4) - dth1*dth4*l2*l4*m4*sin(th3 + th4) - dth2*dth3*l2*l4*m4*sin(th3 + th4) - dth2*dth4*l2*l4*m4*sin(th3 + th4) - dth1*dth5*l1*l5*m5*sin(th2 + th5) - dth3*dth4*l2*l4*m4*sin(th3 + th4) - dth2*dth5*l1*l5*m5*sin(th2 + th5) - dth1*dth2*l1*l2*m2*sin(th2) - 2*dth1*dth2*l1*l2*m3*sin(th2) - 2*dth1*dth2*l1*l2*m4*sin(th2) - 2*dth1*dth2*l1*l2*m5*sin(th2) - dth1*dth3*l2*l3*m3*sin(th3) - 2*dth1*dth3*l2*l3*m4*sin(th3) - dth2*dth3*l2*l3*m3*sin(th3) - 2*dth2*dth3*l2*l3*m4*sin(th3) - dth1*dth4*l3*l4*m4*sin(th4) - dth2*dth4*l3*l4*m4*sin(th4) - dth3*dth4*l3*l4*m4*sin(th4) - dth1*dth5*l2*l5*m5*sin(th5) - dth2*dth5*l2*l5*m5*sin(th5) - dth1*dth2*l1*l4*m4*sin(th2 + th3 + th4) - dth1*dth3*l1*l4*m4*sin(th2 + th3 + th4) - dth1*dth4*l1*l4*m4*sin(th2 + th3 + th4) - dth2*dth3*l1*l4*m4*sin(th2 + th3 + th4) - dth2*dth4*l1*l4*m4*sin(th2 + th3 + th4) - dth3*dth4*l1*l4*m4*sin(th2 + th3 + th4);
CC(2, 1) = (dth1^2*l1*l3*m3*sin(th2 + th3))/2 + dth1^2*l1*l3*m4*sin(th2 + th3) + (dth1^2*l1*l5*m5*sin(th2 + th5))/2 - (dth3^2*l2*l4*m4*sin(th3 + th4))/2 - (dth4^2*l2*l4*m4*sin(th3 + th4))/2 + (dth1^2*l1*l2*m2*sin(th2))/2 + dth1^2*l1*l2*m3*sin(th2) + dth1^2*l1*l2*m4*sin(th2) + dth1^2*l1*l2*m5*sin(th2) - (dth3^2*l2*l3*m3*sin(th3))/2 - dth3^2*l2*l3*m4*sin(th3) - (dth4^2*l3*l4*m4*sin(th4))/2 - (dth5^2*l2*l5*m5*sin(th5))/2 + (dth1^2*l1*l4*m4*sin(th2 + th3 + th4))/2 - dth1*dth3*l2*l4*m4*sin(th3 + th4) - dth1*dth4*l2*l4*m4*sin(th3 + th4) - dth2*dth3*l2*l4*m4*sin(th3 + th4) - dth2*dth4*l2*l4*m4*sin(th3 + th4) - dth3*dth4*l2*l4*m4*sin(th3 + th4) - dth1*dth3*l2*l3*m3*sin(th3) - 2*dth1*dth3*l2*l3*m4*sin(th3) - dth2*dth3*l2*l3*m3*sin(th3) - 2*dth2*dth3*l2*l3*m4*sin(th3) - dth1*dth4*l3*l4*m4*sin(th4) - dth2*dth4*l3*l4*m4*sin(th4) - dth3*dth4*l3*l4*m4*sin(th4) - dth1*dth5*l2*l5*m5*sin(th5) - dth2*dth5*l2*l5*m5*sin(th5);
CC(3, 1) = (dth1^2*l1*l3*m3*sin(th2 + th3))/2 + dth1^2*l1*l3*m4*sin(th2 + th3) + (dth1^2*l2*l4*m4*sin(th3 + th4))/2 + (dth2^2*l2*l4*m4*sin(th3 + th4))/2 + (dth1^2*l2*l3*m3*sin(th3))/2 + dth1^2*l2*l3*m4*sin(th3) + (dth2^2*l2*l3*m3*sin(th3))/2 + dth2^2*l2*l3*m4*sin(th3) - (dth4^2*l3*l4*m4*sin(th4))/2 + (dth1^2*l1*l4*m4*sin(th2 + th3 + th4))/2 + dth1*dth2*l2*l4*m4*sin(th3 + th4) + dth1*dth2*l2*l3*m3*sin(th3) + 2*dth1*dth2*l2*l3*m4*sin(th3) - dth1*dth4*l3*l4*m4*sin(th4) - dth2*dth4*l3*l4*m4*sin(th4) - dth3*dth4*l3*l4*m4*sin(th4);
CC(4, 1) = (l4*m4*(dth1^2*l2*sin(th3 + th4) + dth2^2*l2*sin(th3 + th4) + dth1^2*l3*sin(th4) + dth2^2*l3*sin(th4) + dth3^2*l3*sin(th4) + dth1^2*l1*sin(th2 + th3 + th4) + 2*dth1*dth2*l2*sin(th3 + th4) + 2*dth1*dth2*l3*sin(th4) + 2*dth1*dth3*l3*sin(th4) + 2*dth2*dth3*l3*sin(th4)))/2;
CC(5, 1) = (l5*m5*(dth1^2*l1*sin(th2 + th5) + dth1^2*l2*sin(th5) + dth2^2*l2*sin(th5) + 2*dth1*dth2*l2*sin(th5)))/2;

%% Gravity Vector
GG = zeros(5,1);

GG(1, 1) = (m3*(l2*cos(th1 + th2) + l1*cos(th1) + (l3*cos(th1 + th2 + th3))/2) + m5*(l2*cos(th1 + th2) + l1*cos(th1) + (l5*cos(th1 + th2 + th5))/2) + m2*((l2*cos(th1 + th2))/2 + l1*cos(th1)) + m4*((l4*cos(th1 + th2 + th3 + th4))/2 + l2*cos(th1 + th2) + l1*cos(th1) + l3*cos(th1 + th2 + th3)) + (l1*m1*cos(th1))/2)*gravi;
GG(2, 1) = (m3*(l2*cos(th1 + th2) + (l3*cos(th1 + th2 + th3))/2) + m5*(l2*cos(th1 + th2) + (l5*cos(th1 + th2 + th5))/2) + m4*((l4*cos(th1 + th2 + th3 + th4))/2 + l2*cos(th1 + th2) + l3*cos(th1 + th2 + th3)) + (l2*m2*cos(th1 + th2))/2)*gravi;
GG(3, 1) = (m4*((l4*cos(th1 + th2 + th3 + th4))/2 + l3*cos(th1 + th2 + th3)) + (l3*m3*cos(th1 + th2 + th3))/2)*gravi;
GG(4, 1) = ((l4*m4*cos(th1 + th2 + th3 + th4))/2)*gravi;
GG(5, 1) = ((l5*m5*cos(th1 + th2 + th5))/2)*gravi;

%% input torques mapping matrix
S = [
    1,0,0,0,0;
    0,1,0,0,0;
    0,0,1,0,0;
    0,0,0,1,0;
    0,0,-1,0,1;];

%% Biarticular Spring Force
if sim_settings.use_variable_stiffness_BA
    U_varStiff_BA(isnan(U_varStiff_BA)) = 0; % Convert NaN values to 0

    [tau_st, tau_sw, ~, ~] = calculate_BA_torques( ...
        X, param, U_varStiff_BA);
else
    [tau_st, tau_sw, ~, ~] = calculate_BA_torques( ...
        X, param);
end


%% Constraint Force Calculation (in case of Double Stance)
J_c = zeros(2,5);
J_c(1,1) = - l4*sin(th1 + th2 + th3 + th4) - l3*sin(th1 + th2 + th3) - l2*sin(th1 + th2) - l1*sin(th1);
J_c(1,2) = - l4*sin(th1 + th2 + th3 + th4) - l3*sin(th1 + th2 + th3) - l2*sin(th1 + th2);
J_c(1,3) = - l4*sin(th1 + th2 + th3 + th4) - l3*sin(th1 + th2 + th3);
J_c(1,4) = - l4*sin(th1 + th2 + th3 + th4);
J_c(1,5) = 0;

J_c(2,1) = l4*cos(th1 + th2 + th3 + th4) + l2*cos(th1 + th2) + l1*cos(th1) + l3*cos(th1 + th2 + th3);
J_c(2,2) = l4*cos(th1 + th2 + th3 + th4) + l2*cos(th1 + th2) + l3*cos(th1 + th2 + th3);
J_c(2,3) = l4*cos(th1 + th2 + th3 + th4) + l3*cos(th1 + th2 + th3);
J_c(2,4) = l4*cos(th1 + th2 + th3 + th4);
J_c(2,5) = 0;

dJ_c = zeros(2,5);
dJ_c(1,1) = - dth3*(l4*cos(th1 + th2 + th3 + th4) + l3*cos(th1 + th2 + th3)) - dth1*(l4*cos(th1 + th2 + th3 + th4) + l2*cos(th1 + th2) + l1*cos(th1) + l3*cos(th1 + th2 + th3)) - dth2*(l4*cos(th1 + th2 + th3 + th4) + l2*cos(th1 + th2) + l3*cos(th1 + th2 + th3)) - dth4*l4*cos(th1 + th2 + th3 + th4);
dJ_c(1,2) = - dth3*(l4*cos(th1 + th2 + th3 + th4) + l3*cos(th1 + th2 + th3)) - dth1*(l4*cos(th1 + th2 + th3 + th4) + l2*cos(th1 + th2) + l3*cos(th1 + th2 + th3)) - dth2*(l4*cos(th1 + th2 + th3 + th4) + l2*cos(th1 + th2) + l3*cos(th1 + th2 + th3)) - dth4*l4*cos(th1 + th2 + th3 + th4);
dJ_c(1,3) = - dth1*(l4*cos(th1 + th2 + th3 + th4) + l3*cos(th1 + th2 + th3)) - dth2*(l4*cos(th1 + th2 + th3 + th4) + l3*cos(th1 + th2 + th3)) - dth3*(l4*cos(th1 + th2 + th3 + th4) + l3*cos(th1 + th2 + th3)) - dth4*l4*cos(th1 + th2 + th3 + th4);
dJ_c(1,4) = - l4*cos(th1 + th2 + th3 + th4)*(dth1 + dth2 + dth3 + dth4);
dJ_c(1,5) = 0;

dJ_c(2,1) = - dth2*(l4*sin(th1 + th2 + th3 + th4) + l2*sin(th1 + th2) + l3*sin(th1 + th2 + th3)) - dth3*(l4*sin(th1 + th2 + th3 + th4) + l3*sin(th1 + th2 + th3)) - dth1*(l4*sin(th1 + th2 + th3 + th4) + l2*sin(th1 + th2) + l1*sin(th1) + l3*sin(th1 + th2 + th3)) - dth4*l4*sin(th1 + th2 + th3 + th4);
dJ_c(2,2) = - dth1*(l4*sin(th1 + th2 + th3 + th4) + l2*sin(th1 + th2) + l3*sin(th1 + th2 + th3)) - dth2*(l4*sin(th1 + th2 + th3 + th4) + l2*sin(th1 + th2) + l3*sin(th1 + th2 + th3)) - dth3*(l4*sin(th1 + th2 + th3 + th4) + l3*sin(th1 + th2 + th3)) - dth4*l4*sin(th1 + th2 + th3 + th4);
dJ_c(2,3) = - dth1*(l4*sin(th1 + th2 + th3 + th4) + l3*sin(th1 + th2 + th3)) - dth2*(l4*sin(th1 + th2 + th3 + th4) + l3*sin(th1 + th2 + th3)) - dth3*(l4*sin(th1 + th2 + th3 + th4) + l3*sin(th1 + th2 + th3)) - dth4*l4*sin(th1 + th2 + th3 + th4);
dJ_c(2,4) = - l4*sin(th1 + th2 + th3 + th4)*(dth1 + dth2 + dth3 + dth4);
dJ_c(2,5) = 0;

constraint_force = zeros(2,1);
constraint_force = -inv(J_c*inv(MM)*J_c')*(J_c*inv(MM)*(S*U+tau_sw+tau_st-CC-GG)+dJ_c*dq);

%% Disturbance

flag_dist = f_dist(1);
F_dist_x = f_dist(2);
F_dist_y = f_dist(3);

J_dist = [
    - l2*sin(th1 + th2) - l1*sin(th1), -l2*sin(th1 + th2), 0, 0, 0;
      l2*cos(th1 + th2) + l1*cos(th1),  l2*cos(th1 + th2), 0, 0, 0];

%% Acceleration Calculation
ddq = zeros(5,1);
rec_cs_force = [0;0;0;0];

switch_time = flag(4); % time when double stance phase begins

if flag_dist == 1 && (t >= 10 && t <=10.1)
    % if the disturbance is enabled
    if (f_SS == -1 && constraint_force(2) >= 0) || (f_SS == -1 && t - switch_time < 0.05) % second part is because right after impact, there might be some fluctuations so it disregards them for 0.01 secs
        % if f_SS == 0
        ddq = inv(MM)*(- CC - GG + S*U + tau_sw + tau_st + transpose(J_c)*constraint_force + transpose(J_dist)*[F_dist_x; F_dist_y]);
        rec_cs_force = [constraint_force; 0;0];
    else
        rec_cs_force = [0; 0; constraint_force];
        constraint_force = [0; 0]; % don't constraint the swing foot if force in horizontal direction is pulling if its not right after the impact
        ddq = inv(MM)*(- CC - GG + S*U + tau_sw + tau_st + transpose(J_dist)*[F_dist_x; F_dist_y]);
    end
else
    % if the disturbance is disabled
    if (f_SS == -1 && constraint_force(2) >= 0) || (f_SS == -1 && t - switch_time < 0.05) % second part is because right after impact, there might be some fluctuations so it disregards them for 0.01 secs
        % if f_SS == 0
        ddq = inv(MM)*(- CC - GG + S*U + tau_sw + tau_st + transpose(J_c)*constraint_force);
        rec_cs_force = [constraint_force; 0;0];
    else
        rec_cs_force = [0; 0; constraint_force];
        constraint_force = [0; 0]; % don't constraint the swing foot if force in horizontal direction is pulling if its not right after the impact
        ddq = inv(MM)*(- CC - GG + S*U + tau_sw + tau_st);
    end
end


%% VLO Detection

CoM = calculate_com(X, param, 0, [0;0;0;0;0]); % calculation the CoM location
if CoM(1) >= 0
    flg_VLO = 1;
else
    flg_VLO = 0;
end

%%
dX = [dq; ddq];

end

== matlab function model_5LinkWalking/Model dynamics/STOP system when dx_CoM<=0/MATLAB Function1 ==
  data: X input; param input; flag input; zG output; dxG output; th2 output; th4 output
function [zG, dxG, th2, th4] = fcn(X,param, flag)

%% variables
th1 = X(1);
th2 = X(2);
th3 = X(3);
th4 = X(4);
th5 = X(5);

dth1 = X(6);
dth2 = X(7);
dth3 = X(8);
dth4 = X(9);
dth5 = X(10);

q = [th1;th2;th3;th4;th5];
dq = [dth1;dth2;dth3;dth4;dth5];

%% parameters

m1 = param(1);
m2 = param(2);
m3 = m2;
m4 = m1;
m5 = param(3);

l1 = param(4);
l2 = param(5);
l5 = param(6);
l3 = l2;
l4 = l1;

gravi = param(7);
I1 = param(8);
I2 = param(9);
I5 = param(10);
I3 = I1;
I4 = I2;

k_s = param(11);
r_k = param(12);
r_b = param(13);

%% flags
f_SS = flag(1); % indicates which stance phase it is
foot = flag(2); % location of the stance foot
foot_prev = flag(3); % previous location of the stance foot

%% CoM calculation
% CoM = [xG, zG, dxG, dzG, ddxG, ddzG];
CoM = calculate_com(X, param, 0, [0;0;0;0;0]); % calculation the CoM location

xG = CoM(1);
zG = CoM(2);
dxG = CoM(3);
dzG = CoM(4);
